simulink model "model_1"  (R2018b)
settings: Solver=daessc  StartTime=0.0  StopTime=1  RelTol=1e-3
StopFcn:
  | fault = 0
  | %
  | %
  | %
  | %
  | location = 0
  | %
  | %
  | %
  | %
  | %
  | simout(:,13) = fault;
  | simout(:,14) = location;
  | data = xlsread('E:\Project\Simulation\Second\Pavan\samples');
  | data = [data;simout];
  | xlswrite('E:\Project\Simulation\Second\Pavan\samples',data);
libraries: powerlib x7, powerlib_meascontrol x2
settings Model: Creator=Edagotti Pavankumar  LastModifiedBy=Edagotti Pavankumar
settings SolverCC: ZeroCrossAlgorithm=Adaptive
settings DebuggingCC: IgnoredZcDiagnostic=none

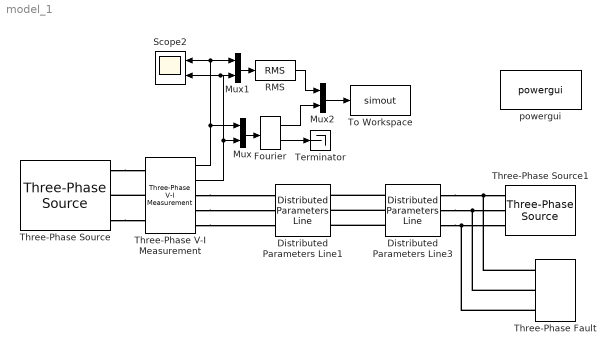
== system model_1 ==
  Distributed Parameters Line1 : powerlib/Elements/Distributed Parameters Line  Phases=3  Frequency=50  Resistance=[0.0238 0.3885]  Inductance=[0.0009509508 0.0032508989]  Capacitance=[12.74e-9 7.751e-9]  Length=150  x1=[5.14282060527251e-10 256106.772031866 256106.772031867;314.159265358979 314.159265358979 314.159265358979;-2.93980542899922 -0.00738555807680356 -1.5781818848717]  x2=[6.16699110845136e-10 257845.414188207 257845.414188208;314.159265358979 314.159265358979 314.159265358979;-3.04146716947045 -0.0331627558342812 -1.60395908262918]  x3=[5.77426137339226e-13 793.939369279763 793.939369279766;314.159265358979 314.159265358979 314.159265358979;2.18585019795315 -0.165205357191776 -1.73600168398668]  x4=[1.30168123336907e-12 1077.72405353391 1077.72405353391;314.159265358979 314.159265358979 314.159265358979;-2.58905380530753 -0.0564897510371113 -1.62728607783201]  x5=0.000752959919858122  V1=[5.143e-10 2.561e+05 2.561e+05;314.2 314.2 314.2;-2.94 -0.007386 -1.578]  V2=[6.167e-10 2.578e+05 2.578e+05;314.2 314.2 314.2;-3.041 -0.03316 -1.604]  I1=[5.774e-13 793.9 793.9;314.2 314.2 314.2;2.186 -0.1652 -1.736]  I2=[1.302e-12 1078 1078;314.2 314.2 314.2;-2.589 -0.05649 -1.627]  nHarmo=1  Measurements=None
      settings: SourceProductName=Simscape Power Systems
  Distributed Parameters Line3 : powerlib/Elements/Distributed Parameters Line  Phases=3  Frequency=50  Resistance=[0.0238 0.3885]  Inductance=[0.0009509508 0.0032508989]  Capacitance=[12.74e-9 7.751e-9]  Length=50  x1=[6.16699110845136e-10 257845.414188207 257845.414188208;314.159265358979 314.159265358979 314.159265358979;-2.88376761262553 0.0761859407649279 -1.49461038602997]  x2=[7.50094417532666e-10 256919.894365681 256919.894365682;314.159265358979 314.159265358979 314.159265358979;-2.90482676997349 0.0680659421058291 -1.50273038468907]  x3=[3.33102165877542e-12 797.604155980678 797.60415598068;314.159265358979 314.159265358979 314.159265358979;2.27883059477739 0.107845420680922 -1.46295090611398]  x4=[3.09591542616291e-12 1083.83935848198 1083.83935848199;314.159265358979 314.159265358979 314.159265358979;-1.75156447269823 -0.00163990961710647 -1.572436236412]  x5=0.000250986639952707  V1=[6.167e-10 2.578e+05 2.578e+05;314.2 314.2 314.2;-2.884 0.07619 -1.495]  V2=[7.501e-10 2.569e+05 2.569e+05;314.2 314.2 314.2;-2.905 0.06807 -1.503]  I1=[3.331e-12 797.6 797.6;314.2 314.2 314.2;2.279 0.1078 -1.463]  I2=[3.096e-12 1084 1084;314.2 314.2 314.2;-1.752 -0.00164 -1.572]  nHarmo=1  Measurements=None
      settings: SourceProductName=Simscape Power Systems
  Fourier : powerlib_meascontrol/Measurements/Fourier  Freq=50  n=1  InInit=[0, 0]  Ts=0
      settings: SourceProductName=Simscape Power Systems
  Mux : Mux  Inputs=2
  Mux1 : Mux  Inputs=2
  Mux2 : Mux  Inputs=2
  RMS : powerlib_meascontrol/Measurements/RMS  TrueRMS=on  Freq=50  RMSInit=0  Ts=0
  Scope2 : Scope  NumInputPorts=2
  Terminator : Terminator
  Three-Phase V-I Measurement : powerlib/Measurements/Three-Phase V-I Measurement  VoltageMeasurement=phase-to-ground  SetLabelV=off  LabelV=Vabc  Vpu=on  VpuLL=off  CurrentMeasurement=yes  SetLabelI=off  LabelI=Iabc  Ipu=on  Pbase=100e6  Vbase=220e3  OutputType=Complex  PhasorSimulation=off  PSBequivalent=0
  Three-Phase Fault : powerlib/Elements/Three-Phase Fault  InitialStates=0  FaultA=on  FaultB=on  FaultC=on  GroundFault=off  SwitchTimes=5  External=off  SwitchStatus=NaN  FaultResistance=20  GroundResistance=0.001  SnubberResistance=1e6  SnubberCapacitance=inf  Measurements=None
  Three-Phase Source : powerlib/Electrical Sources/Three-Phase Source  InternalConnection=Yg  VoltagePhases=off  Voltage=220e3  PhaseAngle=0  Voltage_phases=[25e3 25e3 25e3]/sqrt(3)  PhaseAngles_phases=[0 -120 +120]  Frequency=50  NonIdealSource=on  SpecifyImpedance=on  Resistance=0.8929  Inductance=16.58e-3  ShortCircuitLevel=100e6  BaseVoltage=220e3  XRratio=7  BusType=swing  Pref=10e3  Qref=0  Prefabc=[10e3, 10e3, 10e3]  Qrefabc=[0, 0, 0]  Qmin=-inf  Qmax=inf
  Three-Phase Source1 : powerlib/Electrical Sources/Three-Phase Source  InternalConnection=Yg  VoltagePhases=off  Voltage=220e3  PhaseAngle=-40  Voltage_phases=[25e3 25e3 25e3]/sqrt(3)  PhaseAngles_phases=[0 -120 +120]  Frequency=50  NonIdealSource=on  SpecifyImpedance=on  Resistance=0.8929  Inductance=16.58e-3  ShortCircuitLevel=100e6  BaseVoltage=220e3  XRratio=7  BusType=PV  Pref=inf  Qref=0  Prefabc=[10e3, 10e3, 10e3]  Qrefabc=[0, 0, 0]  Qmin=-inf  Qmax=inf
  To Workspace : ToWorkspace  VariableName=simout  SampleTime=-1
      settings: MaxDataPoints=200  Save2DSignal=2-D array (concatenate along first dimension)
  powergui : powerlib/powergui  Priority=1  SimulationMode=Continuous  SampleTime=50e-10  frequency=60  Iterations=50  frequencyindice=50  Pbase=100e6  ErrMax=1e-4  UnitsV=kV  UnitsW=MW  buscounter=0  FunctionMessages=off  echomessages=off  EnableUseOfTLC=off  CurrentSourceSwitches=off  DisableSnubberDevices=off  DisableRonSwitches=off  DisableVfSwitches=off  DisplayEquations=off  SolverType=Tustin/Backward Euler (TBE)  Interpol=off  ExternalGateDelay=off  methode=off  Ts=100  x0status=blocks  SPID=off  SwTol=0  HookPort=off  RestoreLinks=warning  ResistiveCurrentMeasurement=off  Frange=[0:2:500]  Ylog=off  Xlog=on  ShowGrid=off  save=off  variable=ZData  structure=0  ZoomFFT=off  StartTime=0.0  cycles=1  DisplayStyle=1  fundamental=60  FreqAxis=off  MaxFrequency=1000  frequencyindicesteady=1  RmsSteady=2  display=off
  wires:
  Fourier/1 -> Terminator/1
  Mux/1 -> Fourier/1
  Mux2/1 -> To Workspace/1
  Three-Phase V-I Measurement/2 -> Mux/2, Scope2/2, Mux1/2
  RMS/1 -> Mux2/1
  Three-Phase V-I Measurement/1 -> Mux/1, Mux1/1, Scope2/1
  Mux1/1 -> RMS/1
  Fourier/2 -> Mux2/2
  connections:
  Three-Phase V-I Measurement/RConn2 -- Distributed Parameters Line1/LConn2
  Three-Phase V-I Measurement/RConn1 -- Distributed Parameters Line1/LConn1
  Three-Phase V-I Measurement/RConn3 -- Distributed Parameters Line1/LConn3
  Three-Phase Source/RConn1 -- Three-Phase V-I Measurement/LConn1
  Distributed Parameters Line3/RConn1 -- Three-Phase Fault/LConn1 -- Three-Phase Source1/RConn1
  Distributed Parameters Line3/LConn2 -- Distributed Parameters Line1/RConn2
  Distributed Parameters Line3/RConn2 -- Three-Phase Fault/LConn2 -- Three-Phase Source1/RConn2
  Three-Phase Source/RConn3 -- Three-Phase V-I Measurement/LConn3
  Distributed Parameters Line3/LConn3 -- Distributed Parameters Line1/RConn3
  Three-Phase V-I Measurement/LConn2 -- Three-Phase Source/RConn2
  Distributed Parameters Line3/RConn3 -- Three-Phase Fault/LConn3 -- Three-Phase Source1/RConn3
  Distributed Parameters Line3/LConn1 -- Distributed Parameters Line1/RConn1
